simulink model "sampleModel281"  (R2021b)
settings: Solver=VariableStepAuto  StartTime=0.0  StopTime=10.0  RelTol=1e-3
undefined symbols (not defined in the file or in its folder): Newton, Raphson
libraries: simulink x13, slpidlib x3
settings Model: Creator=user  LastModifiedBy=user

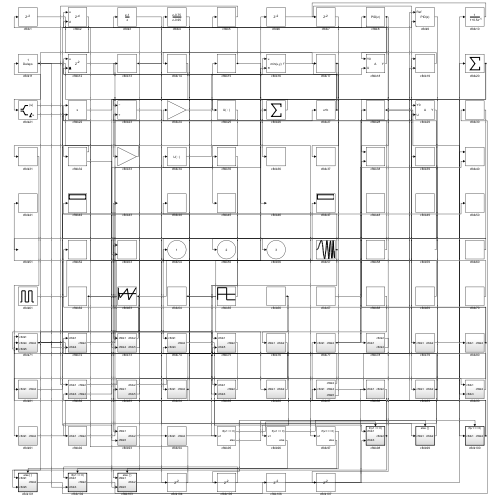
[thumbnail: Simulink's stored preview of the top-level diagram]
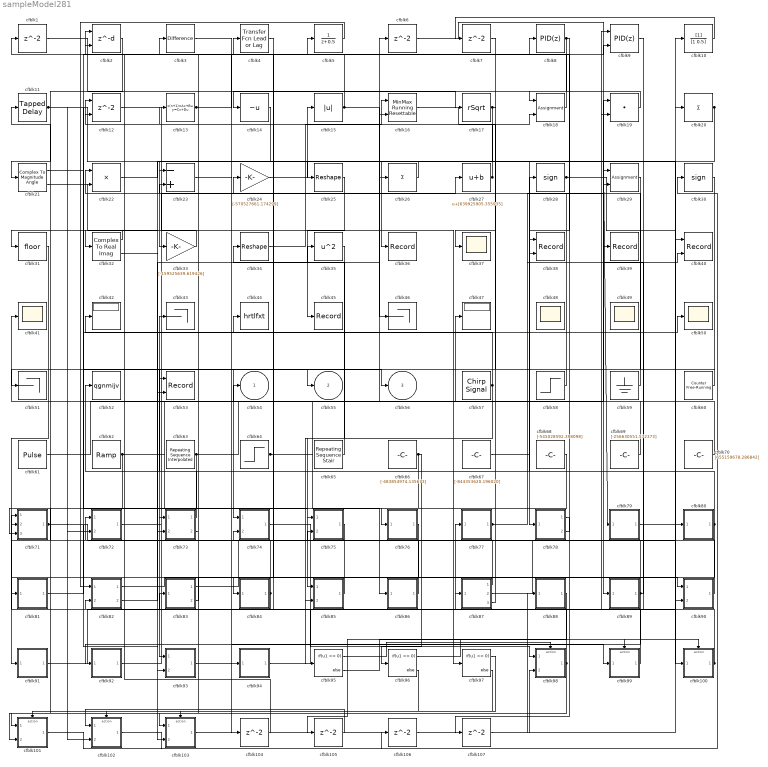
== system sampleModel281 ==
  cfblk{1,6..7,104..107} (7 alike) : Delay  SampleTime=1
  cfblk10 : DiscreteFilter  SampleTime=1
  cfblk100 : Subsystem  TreatAsAtomicUnit=on
  cfblk101 : Subsystem  TreatAsAtomicUnit=on
  cfblk102 : Subsystem  TreatAsAtomicUnit=on
  cfblk103 : Subsystem  TreatAsAtomicUnit=on
  cfblk11 : simulink/Discrete/Tapped Delay  vinit=0.0  samptime=-1  NumDelays=1  DelayOrder=Oldest  includeCurrent=off
  cfblk12 : Delay  ShowEnablePort=on  SampleTime=1
      settings: InputPortMap=u0,e6
  cfblk13 : DiscreteStateSpace
  cfblk14 : UnaryMinus
  cfblk15 : Abs
  cfblk16 : simulink/Math Operations/MinMax Running Resettable  Function=min  vinit=0.0
  cfblk17 : Sqrt  Operator=rSqrt  AlgorithmType=Newton-Raphson  SaturateOnIntegerOverflow=on
  cfblk18 : Assignment  DiagnosticForDimensions=Warning  IndexOptions=Index vector (dialog)  Indices=1  OutputSizes=1
  cfblk19 : DotProduct  InputSameDT=on  OutDataTypeStr=Inherit: Inherit via internal rule
  cfblk2 : Delay  DelayLengthSource=Input port  SampleTime=1
      settings: InputPortMap=u0,p1
  cfblk20 : Sum  Inputs=+
  cfblk21 : ComplexToMagnitudeAngle
  cfblk22 : Product  Inputs=**
  cfblk23 : Sum  Inputs=-+
  cfblk24 : Gain  Gain=[-570527661.174299]
  cfblk25 : Reshape
  cfblk26 : Sum  Inputs=+
  cfblk27 : Bias  Bias=[639925905.355935]
  cfblk28 : Signum
  cfblk29 : Assignment  DiagnosticForDimensions=Warning  IndexOptions=Index vector (dialog)  Indices=1  OutputSizes=1
  cfblk3 : simulink/Discrete/Difference  ICPrevInput=0.0  OutMin=[]  OutMax=[]  OutDataTypeStr=Inherit: Inherit via back propagation  OutDataType=fixdt(1, 16)  OutScaling=2^-10  DoSatur=off
  cfblk30 : Signum
  cfblk31 : Rounding
  cfblk32 : ComplexToRealImag
  cfblk33 : Gain  Gain=[-159525639.619426]
  cfblk34 : Reshape
  cfblk35 : Math  Operator=square  SaturateOnIntegerOverflow=on
  cfblk36 : Record  FileSettingsInternal="{\"entries\":[{\"content\":{\"excelSettings\":{\"content\":{},\"type\":\"Streamout.ExcelSettings\"}},\"type\":\"Streamout.FileSettingStorage\",\"uuid\":\"c781cdf7-8340-408b-8422-f8d69e560093\"}],\"packageUris\":[\"http://schema.mathworks.com/mf0/streamout_blocks/R2020a\"],\"version\":\"1.0\"}"  SignalsInternal="{\"entries\":[{\"content\":{\"signals\":[{\"content\":{\"blockPath\":[\"sampleModel281/cfblk36\"],\"channel\":[],\"dimensions\":[1],\"domain\":\"sampleModel281/cfblk36\",\"lineColor\":\"#139fff\",\"plots\":[1],\"port\":1,\"sid\":[\"\"],\"signalID\":11991,\"signalName\":\"cfblk17\"},\"type\":\"RecordBlkView.Signal\",\"uuid\":\"6f29a3cb-49ad-40a3-998c-ead64aca4211\"}]},\"type\":\"RecordBlkView.InputSignals\",\"uuid\":\"da20b184-1727-445b-b2e6-5f57a6227382\"}],\"packageUris\":[\"http://schema.mathworks.com/mf0/streamout_blocks/R2020a\"],\"version\":\"1.0\"}"  VisualizationBindings="{\"sparklinesplugin\":{\"info\":[{\"bindingParametersList\":[],\"subplotID\":1}]}}"
  cfblk{37,41,48..50} (5 alike) : Scope
      cfblk48 settings: Floating=on
      cfblk49 settings: Floating=on
  cfblk38 : Record  FileSettingsInternal="{\"entries\":[{\"content\":{\"excelSettings\":{\"content\":{},\"type\":\"Streamout.ExcelSettings\"}},\"type\":\"Streamout.FileSettingStorage\",\"uuid\":\"4188593c-7763-4c79-a663-ea53f92952dd\"}],\"packageUris\":[\"http://schema.mathworks.com/mf0/streamout_blocks/R2020a\"],\"version\":\"1.0\"}"  Layout=[1 1]  SignalsInternal="{\"entries\":[{\"content\":{\"signals\":[{\"content\":{\"blockPath\":[\"sampleModel281/cfblk38\"],\"channel\":[],\"dimensions\":[1],\"domain\":\"sampleModel281/cfblk38\",\"lineColor\":\"#a2142f\",\"plots\":[1],\"port\":1,\"sid\":[\"\"],\"signalID\":11963,\"signalName\":\"cfblk8\"},\"type\":\"RecordBlkView.Signal\",\"uuid\":\"ce15c6e9-b25a-4a9d-a87d-16814ede9b87\"},{\"content\":{\"blockPath\":[\"sampleModel281/cfblk38\"],\"channel\":[],\"dimensions\":[1],\"domain\":\"sampleModel281/cfblk38\",\"lineColor\":\"#139fff\",\"plots\":[1],\"port\":2,\"sid\":[\"\"],\"signalID\":11967,\"signalName\":\"cfblk80\"},\"type\":\"RecordBlkView.Signal\",\"uuid\":\"4c2adb0f-b2cf-481c-9f3f-668d91455d88\"}]},\"type\":\"RecordBlkView.InputSignals\",\"uuid\":\"ebf02ba3-550e-4026-a02e-bf4ccdc05b99\"}],\"packageUris\":[\"http://schema.mathworks.com/mf0/streamout_blocks/R2020a\"],\"version\":\"1.0\"}"  VisualizationBindings="{\"xyplotplugin\":{\"info\":[{\"series\":[{\"bindingParametersList\":[{\"parameter\":\"X-Axis\",\"signalID\":11963,\"signalName\":\"cfblk8\"},{\"parameter\":\"Y-Axis\",\"signalID\":11967,\"signalName\":\"cfblk80\"}],\"seriesID\":6983}],\"subplotID\":1}]}}"  CompatibilityTag=XY
  cfblk39 : Record  FileSettingsInternal="{\"entries\":[{\"content\":{\"excelSettings\":{\"content\":{},\"type\":\"Streamout.ExcelSettings\"}},\"type\":\"Streamout.FileSettingStorage\",\"uuid\":\"219db649-d65c-4cc3-812d-aced4d92e676\"}],\"packageUris\":[\"http://schema.mathworks.com/mf0/streamout_blocks/R2020a\"],\"version\":\"1.0\"}"  SignalsInternal="{\"entries\":[{\"content\":{\"signals\":[{\"content\":{\"blockPath\":[\"sampleModel281/cfblk39\"],\"channel\":[],\"dimensions\":[1],\"domain\":\"sampleModel281/cfblk39\",\"lineColor\":\"#edb120\",\"plots\":[1],\"port\":1,\"sid\":[\"\"],\"signalID\":11971,\"signalName\":\"cfblk89\"},\"type\":\"RecordBlkView.Signal\",\"uuid\":\"55bd96a2-e860-4ecd-af7d-bb83553d0170\"}]},\"type\":\"RecordBlkView.InputSignals\",\"uuid\":\"8836e843-c683-4200-9918-d583b1163d7b\"}],\"packageUris\":[\"http://schema.mathworks.com/mf0/streamout_blocks/R2020a\"],\"version\":\"1.0\"}"  VisualizationBindings="{\"sparklinesplugin\":{\"info\":[{\"bindingParametersList\":[],\"subplotID\":1}]}}"
  cfblk4 : simulink/Discrete/Transfer Fcn Lead or Lag  PoleZ=0.95  ZeroZ=0.75  ICPrevOutput=0.0  ICPrevInput=0.0  DoSatur=off
      settings: SourceProductBaseCode=SL
  cfblk40 : Record  FileSettingsInternal="{\"entries\":[{\"content\":{\"excelSettings\":{\"content\":{},\"type\":\"Streamout.ExcelSettings\"}},\"type\":\"Streamout.FileSettingStorage\",\"uuid\":\"7e2a92c3-6fd6-43f3-bb8d-8e942b6776ba\"}],\"packageUris\":[\"http://schema.mathworks.com/mf0/streamout_blocks/R2020a\"],\"version\":\"1.0\"}"  Layout=[1 1]  SignalsInternal="{\"entries\":[{\"content\":{\"signals\":[{\"content\":{\"blockPath\":[\"sampleModel281/cfblk40\"],\"channel\":[],\"dimensions\":[1],\"domain\":\"sampleModel281/cfblk40\",\"lineColor\":\"#a2142f\",\"plots\":[1],\"port\":1,\"sid\":[\"\"],\"signalID\":11975,\"signalName\":\"cfblk91\"},\"type\":\"RecordBlkView.Signal\",\"uuid\":\"8dd85c33-c0e1-47fe-82f9-e8373d55203a\"},{\"content\":{\"blockPath\":[\"sampleModel281/cfblk40\"],\"channel\":[],\"dimensions\":[1],\"domain\":\"sampleModel281/cfblk40\",\"lineColor\":\"#139fff\",\"plots\":[1],\"port\":2,\"sid\":[\"\"],\"signalID\":11979,\"signalName\":\"cfblk77\"},\"type\":\"RecordBlkView.Signal\",\"uuid\":\"2f79c080-1485-4a3a-9cf0-de9ca85e6d7b\"}]},\"type\":\"RecordBlkView.InputSignals\",\"uuid\":\"15f4dd09-4716-4c1b-9d4f-630d21f687a7\"}],\"packageUris\":[\"http://schema.mathworks.com/mf0/streamout_blocks/R2020a\"],\"version\":\"1.0\"}"  VisualizationBindings="{\"xyplotplugin\":{\"info\":[{\"series\":[{\"bindingParametersList\":[{\"parameter\":\"X-Axis\",\"signalID\":11975,\"signalName\":\"cfblk91\"},{\"parameter\":\"Y-Axis\",\"signalID\":11979,\"signalName\":\"cfblk77\"}],\"seriesID\":59243}],\"subplotID\":1}]}}"  CompatibilityTag=XY
  cfblk42 : Display
  cfblk43 : Terminator
  cfblk44 : ToWorkspace  VariableName=hrtlfxt  SaveFormat=Timeseries  SampleTime=-1
  cfblk45 : Record  FileSettingsInternal="{\"entries\":[{\"content\":{\"excelSettings\":{\"content\":{},\"type\":\"Streamout.ExcelSettings\"}},\"type\":\"Streamout.FileSettingStorage\",\"uuid\":\"80b63704-7d10-486e-b387-18bfb6728c18\"}],\"packageUris\":[\"http://schema.mathworks.com/mf0/streamout_blocks/R2020a\"],\"version\":\"1.0\"}"  SignalsInternal="{\"entries\":[{\"content\":{\"signals\":[{\"content\":{\"blockPath\":[\"sampleModel281/cfblk45\"],\"channel\":[],\"dimensions\":[1],\"domain\":\"sampleModel281/cfblk45\",\"lineColor\":\"#ff6929\",\"plots\":[1],\"port\":1,\"sid\":[\"\"],\"signalID\":11995,\"signalName\":\"cfblk25\"},\"type\":\"RecordBlkView.Signal\",\"uuid\":\"f8ece178-e086-4969-b784-ed276f630d12\"}]},\"type\":\"RecordBlkView.InputSignals\",\"uuid\":\"7be7d227-b162-4c4c-ad33-f79b945d64e0\"}],\"packageUris\":[\"http://schema.mathworks.com/mf0/streamout_blocks/R2020a\"],\"version\":\"1.0\"}"  VisualizationBindings="{\"sparklinesplugin\":{\"info\":[{\"bindingParametersList\":[],\"subplotID\":1}]}}"
  cfblk46 : Terminator
  cfblk47 : Display
  cfblk5 : DiscreteTransferFcn  SampleTime=1
  cfblk51 : Terminator
  cfblk52 : ToWorkspace  VariableName=qgnmijv  SaveFormat=Timeseries  SampleTime=-1
  cfblk53 : Record  FileSettingsInternal="{\"entries\":[{\"content\":{\"excelSettings\":{\"content\":{},\"type\":\"Streamout.ExcelSettings\"}},\"type\":\"Streamout.FileSettingStorage\",\"uuid\":\"979e6c69-9637-4301-9808-cdf47ec4f26d\"}],\"packageUris\":[\"http://schema.mathworks.com/mf0/streamout_blocks/R2020a\"],\"version\":\"1.0\"}"  Layout=[1 1]  SignalsInternal="{\"entries\":[{\"content\":{\"signals\":[{\"content\":{\"blockPath\":[\"sampleModel281/cfblk53\"],\"channel\":[],\"dimensions\":[1],\"domain\":\"sampleModel281/cfblk53\",\"lineColor\":\"#a2142f\",\"plots\":[1],\"port\":1,\"sid\":[\"\"],\"signalID\":11983,\"signalName\":\"cfblk86\"},\"type\":\"RecordBlkView.Signal\",\"uuid\":\"a6416475-d9fb-464a-9363-37660f0059bb\"},{\"content\":{\"blockPath\":[\"sampleModel281/cfblk53\"],\"channel\":[],\"dimensions\":[1],\"domain\":\"sampleModel281/cfblk53\",\"lineColor\":\"#139fff\",\"plots\":[1],\"port\":2,\"sid\":[\"\"],\"signalID\":11987,\"signalName\":\"cfblk21:2\"},\"type\":\"RecordBlkView.Signal\",\"uuid\":\"573ba67e-6b02-4113-b266-649fc294594e\"}]},\"type\":\"RecordBlkView.InputSignals\",\"uuid\":\"a6bf4982-741b-4a82-8cf7-86aa072de18b\"}],\"packageUris\":[\"http://schema.mathworks.com/mf0/streamout_blocks/R2020a\"],\"version\":\"1.0\"}"  VisualizationBindings="{\"xyplotplugin\":{\"info\":[{\"series\":[{\"bindingParametersList\":[{\"parameter\":\"X-Axis\",\"signalID\":11983,\"signalName\":\"cfblk86\"},{\"parameter\":\"Y-Axis\",\"signalID\":11987,\"signalName\":\"cfblk21:2\"}],\"seriesID\":45068}],\"subplotID\":1}]}}"  CompatibilityTag=XY
  cfblk57 : simulink/Sources/Chirp Signal  f1=[-334643469.224714]  T=[-94135203.309986]  f2=[152847106.360706]
  cfblk58 : Step  Time=[42.000000]  Before=[-159427746.311310]  After=[840646586.279118]  SampleTime=0
  cfblk59 : Ground
  cfblk60 : simulink/Sources/Counter Free-Running  NumBits=[16.000000]  tsamp=-1
  cfblk61 : DiscretePulseGenerator  PulseType=Time based  Amplitude=[-599555559.374941]  Period=[82024512.109082]  PulseWidth=5  PhaseDelay=[9.000000]
  cfblk62 : simulink/Sources/Ramp  slope=[-4599.343733]  start=[27.677113]  InitialOutput=[-405546.025741]
  cfblk63 : simulink/Sources/Repeating Sequence Interpolated  OutValues=[236426282.621736, -510010552.768380, 614187584.766331, -765152925.585290, 735747006.586161]  TimeValues=[0 0.1 0.5 0.6 1].'  LookUpMeth=Use Input Below  tsamp=0.01  OutMin=[]  OutMax=[]  OutDataTypeStr=double  OutputDataTypeScalingMode=double  OutDataType=fixdt(0,8)  OutScaling=2^-10
  cfblk64 : Step  Time=[34.000000]  Before=[-566169938.934532]  After=[306635443.375634]  SampleTime=0
  cfblk65 : simulink/Sources/Repeating Sequence Stair  OutValues=[982481802.198341, -856880890.360256]  tsamp=-1  OutMin=[]  OutMax=[]  OutDataTypeStr=double  OutputDataTypeScalingMode=double  OutDataType=fixdt(0,8)  ConRadixGroup=Best Precision: Vector-wise  OutScaling=2^-12
  cfblk66 : Constant  Value=[-483854974.135673]  SampleTime=1
  cfblk67 : Constant  Value=[-844353620.196020]  SampleTime=1
  cfblk68 : Constant  Value=[-545028592.398098]  SampleTime=1
  cfblk69 : Constant  Value=[-256630551.572373]  SampleTime=1
  cfblk70 : Constant  Value=[655159678.286842]  SampleTime=1
  cfblk71 : Subsystem
  cfblk72 : Subsystem
  cfblk73 : Subsystem
  cfblk74 : Subsystem
  cfblk75 : Subsystem
  cfblk76 : Subsystem
  cfblk77 : Subsystem
  cfblk78 : Subsystem
  cfblk79 : Subsystem
  cfblk8 : slpidlib/PID Controller  Controller=PID  Form=Parallel  TimeDomain=Discrete-time  UseExternalTs=off  SampleTime=1  IntegratorMethod=Forward Euler  FilterMethod=Forward Euler  ControllerParametersSource=internal  P=1  I=1  D=0  UseFilter=on  N=100  TunerSelectOption=Transfer Function Based (PID Tuner App)  InitialConditionSource=internal  InitialConditionForIntegrator=0  InitialConditionForFilter=0  DifferentiatorICPrevScaledInput=0  ExternalReset=none  TrackingMode=off  Kt=1  LimitOutput=off  SatLimitsSource=internal  UpperSaturationLimit=inf  LowerSaturationLimit=-inf  LinearizeAsGain=off  AntiWindupMode=none  Kb=1  POutMin=[]  POutMax=[]  IOutMin=[]  IOutMax=[]  DOutMin=[]  DOutMax=[]  NOutMin=[]  NOutMax=[]  SumOutMin=[]  SumOutMax=[]  SaturationOutMin=[]  SaturationOutMax=[]  PParamMin=[]  PParamMax=[]  IParamMin=[]  IParamMax=[]  DParamMin=[]  DParamMax=[]  NParamMin=[]  NParamMax=[]  KbParamMin=[]  KbParamMax=[]  KtParamMin=[]  KtParamMax=[]  KbOutMin=[]  KbOutMax=[]  KtOutMin=[]  KtOutMax=[]  IntegratorOutMin=[]  IntegratorOutMax=[]  FilterOutMin=[]  FilterOutMax=[]  SumI1OutMin=[]  SumI1OutMax=[]  SumI2OutMin=[]  SumI2OutMax=[]  SumI3OutMin=[]  SumI3OutMax=[]  SumI4OutMin=[]  SumI4OutMax=[]  SumDOutMin=[]  SumDOutMax=[]  DifferentiatorOutMin=[]  DifferentiatorOutMax=[]  FilterDiffOutCoefMin=[]  FilterDiffOutCoefMax=[]  ReciprocalOutMin=[]  ReciprocalOutMax=[]  SumDenOutMin=[]  SumDenOutMax=[]  SumNumOutMin=[]  SumNumOutMax=[]  DivideOutMin=[]  DivideOutMax=[]  UdiffTsProdOutMin=[]  UdiffTsProdOutMax=[]  NTsProdOutMin=[]  NTsProdOutMax=[]  UintegralTsProdOutMin=[]  UintegralTsProdOutMax=[]  UngainTsProdOutMin=[]  UngainTsProdOutMax=[]  IntegratorContinuousStateAttributes=''  IntegratorStateMustResolveToSignalObject=off  IntegratorRTWStateStorageClass=Auto  FilterContinuousStateAttributes=''  FilterStateMustResolveToSignalObject=off  FilterRTWStateStorageClass=Auto  ParallelPVariant=InternalParameters  IdealPVariant=Disabled  IVariant=InternalParameters  DVariant=InternalParameters  IntegratorVariant=Discrete  SatVariant=Disabled  AWVariant=Passthrough  PCopyVariant=Disabled  TRVariant=Disabled  FdbkBlocksVariant=Forward  IdealPFdbkVariant=Disabled  SatFdbkVariant=Disabled  DerivativeFilterVariant=ForwardEulerFilter  NVariant=InternalParameters  NCopyVariant=Disabled  FilterICVariant=InternalICsFilter  IntegratorICVariant=InternalICs  ExternalResetVariant=Disabled  TRSumVariant=Passthrough  SumFdbkVariant=Disabled  SumVariant=Sum_PID  TsampFilterVariant=InternalTs  TsampNgainVariant=Passthrough  TsampIntegralVariant=Passthrough  ExternalSaturationOutDataTypeStr=Inherit: Same as second input
  cfblk80 : Subsystem
  cfblk81 : Subsystem
  cfblk82 : Subsystem
  cfblk83 : Subsystem
  cfblk84 : Subsystem
  cfblk85 : Subsystem
  cfblk86 : Subsystem
  cfblk87 : Subsystem
  cfblk88 : Subsystem
  cfblk89 : Subsystem
  cfblk9 : slpidlib/PID Controller (2DOF)  Controller=PID  Form=Parallel  TimeDomain=Discrete-time  UseExternalTs=off  SampleTime=1  IntegratorMethod=Forward Euler  FilterMethod=Forward Euler  ControllerParametersSource=internal  P=1  I=1  D=0  UseFilter=on  N=100  b=1  c=1  TunerSelectOption=Transfer Function Based (PID Tuner App)  InitialConditionSource=internal  InitialConditionForIntegrator=0  InitialConditionForFilter=0  DifferentiatorICPrevScaledInput=0  ExternalReset=none  TrackingMode=off  Kt=1  LimitOutput=off  SatLimitsSource=internal  UpperSaturationLimit=inf  LowerSaturationLimit=-inf  LinearizeAsGain=off  AntiWindupMode=none  Kb=1  POutMin=[]  POutMax=[]  IOutMin=[]  IOutMax=[]  DOutMin=[]  DOutMax=[]  NOutMin=[]  NOutMax=[]  bOutMin=[]  bOutMax=[]  cOutMin=[]  cOutMax=[]  SumOutMin=[]  SumOutMax=[]  SaturationOutMin=[]  SaturationOutMax=[]  PParamMin=[]  PParamMax=[]  IParamMin=[]  IParamMax=[]  DParamMin=[]  DParamMax=[]  NParamMin=[]  NParamMax=[]  bParamMin=[]  bParamMax=[]  cParamMin=[]  cParamMax=[]  KbParamMin=[]  KbParamMax=[]  KtParamMin=[]  KtParamMax=[]  KbOutMin=[]  KbOutMax=[]  KtOutMin=[]  KtOutMax=[]  IntegratorOutMin=[]  IntegratorOutMax=[]  FilterOutMin=[]  FilterOutMax=[]  SumI1OutMin=[]  SumI1OutMax=[]  SumI2OutMin=[]  SumI2OutMax=[]  SumI3OutMin=[]  SumI3OutMax=[]  SumI4OutMin=[]  SumI4OutMax=[]  SumDOutMin=[]  SumDOutMax=[]  Sum1OutMin=[]  Sum1OutMax=[]  Sum2OutMin=[]  Sum2OutMax=[]  Sum3OutMin=[]  Sum3OutMax=[]  DifferentiatorOutMin=[]  DifferentiatorOutMax=[]  FilterDiffOutCoefMin=[]  FilterDiffOutCoefMax=[]  ReciprocalOutMin=[]  ReciprocalOutMax=[]  SumDenOutMin=[]  SumDenOutMax=[]  SumNumOutMin=[]  SumNumOutMax=[]  DivideOutMin=[]  DivideOutMax=[]  UdiffTsProdOutMin=[]  UdiffTsProdOutMax=[]  NTsProdOutMin=[]  NTsProdOutMax=[]  UintegralTsProdOutMin=[]  UintegralTsProdOutMax=[]  UngainTsProdOutMin=[]  UngainTsProdOutMax=[]  IntegratorContinuousStateAttributes=''  IntegratorStateMustResolveToSignalObject=off  IntegratorRTWStateStorageClass=Auto  FilterContinuousStateAttributes=''  FilterStateMustResolveToSignalObject=off  FilterRTWStateStorageClass=Auto  ParallelPVariant=InternalParameters  IdealPVariant=Disabled  IVariant=InternalParameters  DVariant=InternalParameters  bVariant=InternalParameters  cVariant=InternalParameters  IntegratorVariant=Discrete  SatVariant=Disabled  AWVariant=Passthrough  PCopyVariant=Disabled  TRVariant=Disabled  FdbkBlocksVariant=Forward  IdealPFdbkVariant=Disabled  SatFdbkVariant=Disabled  DerivativeFilterVariant=ForwardEulerFilter  NVariant=InternalParameters  NCopyVariant=Disabled  FilterICVariant=InternalICsFilter  IntegratorICVariant=InternalICs  ExternalResetVariant=Disabled  TRSumVariant=Passthrough  SumFdbkVariant=Disabled  SumVariant=Sum_PID  TsampFilterVariant=InternalTs  TsampNgainVariant=Passthrough  TsampIntegralVariant=Passthrough  ExternalSaturationOutDataTypeStr=Inherit: Same as second input
      settings: SourceProductBaseCode=SL
  cfblk90 : Subsystem
  cfblk91 : Subsystem
  cfblk92 : Subsystem
  cfblk93 : Subsystem
  cfblk94 : Subsystem
  cfblk95 : If  IfExpression=u1 >= 0  SampleTime=1
  cfblk96 : If  IfExpression=u1 >= 0  SampleTime=1
  cfblk97 : If  IfExpression=u1 >= 0  SampleTime=1
  cfblk98 : Subsystem  TreatAsAtomicUnit=on
  cfblk99 : Subsystem  TreatAsAtomicUnit=on
  cfblk54 : Outport
  cfblk55 : Outport  Port=2
  cfblk56 : Outport  Port=3
  wires:
  cfblk92/1(cfblk2) -> cfblk27/1
  cfblk7/1 -> cfblk55/1
  cfblk17/1 -> cfblk36/1, cfblk37/1
  cfblk14/1 -> cfblk33/1
  cfblk58/1 -> cfblk24/1
  cfblk57/1 -> cfblk42/1, cfblk85/2(cfblk3)
  cfblk6/1 -> cfblk89/1(cfblk1)
  cfblk72/1(cfblk2) -> cfblk26/1
  cfblk65/1 -> cfblk4/1
  cfblk76/1(cfblk2) -> cfblk103/1(cfblk1)
  cfblk9/1 -> cfblk77/1(cfblk1)
  cfblk4/1 -> cfblk84/1(cfblk1)
  cfblk31/1 -> cfblk91/1(cfblk1)
  cfblk25/1 -> cfblk45/1
  cfblk19/1 -> cfblk18/1
  cfblk29/1 -> cfblk74/1(cfblk1)
  cfblk33/1 -> cfblk32/1
  cfblk100/1(cfblk2) -> cfblk54/1, cfblk71/2(cfblk4)
  cfblk28/1 -> cfblk79/1(cfblk1), cfblk90/2(cfblk3)
  cfblk5/1 -> cfblk82/1(cfblk1)
  cfblk70/1 -> cfblk41/1
  cfblk66/1 -> cfblk76/1(cfblk1), cfblk96/1
  cfblk20/1 -> cfblk78/1(cfblk1), cfblk103/2(cfblk5)
  cfblk60/1 -> cfblk51/1
  cfblk16/1 -> cfblk18/2
  cfblk75/1(cfblk2) -> cfblk74/2(cfblk3)
  cfblk8/1 -> cfblk14/1, cfblk38/1
  cfblk102/1(cfblk2) -> cfblk30/1
  cfblk12/1 -> cfblk97/1
  cfblk74/1(cfblk2) -> cfblk98/1(cfblk1)
  cfblk30/1 -> cfblk93/1(cfblk1)
  cfblk98/1(cfblk2) -> cfblk87/1(cfblk1), cfblk101/2(cfblk5)
  cfblk87/1(cfblk2) -> cfblk44/1
  cfblk68/1 -> cfblk73/1(cfblk1)
  cfblk26/1 -> cfblk23/1
  cfblk35/1 -> cfblk85/1(cfblk1)
  cfblk61/1 -> cfblk19/1
  cfblk90/1(cfblk2) -> cfblk11/1
  cfblk15/1 -> cfblk46/1, cfblk1/1
  cfblk1/1 -> cfblk17/1
  cfblk82/1(cfblk2) -> cfblk90/1(cfblk1)
  cfblk80/1(cfblk2) -> cfblk52/1, cfblk38/2, cfblk81/1(cfblk1)
  cfblk69/1 -> cfblk22/1
  cfblk73/1(cfblk2) -> cfblk43/1
  cfblk84/1(cfblk2) -> cfblk13/1, cfblk82/2(cfblk3)
  cfblk86/1(cfblk2) -> cfblk53/1
  cfblk11/1 -> cfblk100/1(cfblk1), cfblk72/2(cfblk4), cfblk56/1
  cfblk87/2(cfblk4) -> cfblk10/1
  cfblk73/2(cfblk5) -> cfblk23/2
  cfblk2/1 -> cfblk21/1
  cfblk23/1 -> cfblk94/1(cfblk1)
  cfblk89/1(cfblk2) -> cfblk39/1, cfblk34/1, cfblk92/1(cfblk1)
  cfblk18/1 -> cfblk2/1
  cfblk10/1 -> cfblk7/1
  cfblk64/1 -> cfblk86/1(cfblk1), cfblk47/1
  cfblk24/1 -> cfblk15/1
  cfblk79/1(cfblk2) -> cfblk80/1(cfblk1)
  cfblk99/1(cfblk2) -> cfblk83/1(cfblk1)
  cfblk83/1(cfblk2) -> cfblk9/1
  cfblk94/1(cfblk2) -> cfblk19/2
  cfblk21/1 -> cfblk75/1(cfblk1)
  cfblk3/1 -> cfblk99/1(cfblk1)
  cfblk82/2(cfblk4) -> cfblk35/1
  cfblk34/1 -> cfblk16/1
  cfblk71/1(cfblk2) -> cfblk75/2(cfblk5), cfblk93/2(cfblk5), cfblk102/2(cfblk3), cfblk50/1
  cfblk85/1(cfblk2) -> cfblk71/1(cfblk1)
  cfblk103/1(cfblk2) -> cfblk88/1(cfblk1)
  cfblk62/1 -> cfblk95/1, cfblk16/2, cfblk101/1(cfblk1)
  cfblk22/1 -> cfblk25/1
  cfblk81/1(cfblk2) -> cfblk8/1
  cfblk83/2(cfblk5) -> cfblk72/1(cfblk1)
  cfblk21/2 -> cfblk53/2
  cfblk63/1 -> cfblk6/1, cfblk71/3(cfblk5)
  cfblk91/1(cfblk2) -> cfblk40/1
  cfblk13/1 -> cfblk9/2, cfblk29/1
  cfblk87/3(cfblk5) -> cfblk12/1
  cfblk78/2(cfblk4) -> cfblk5/1
  cfblk67/1 -> cfblk28/1
  cfblk27/1 -> cfblk12/2, cfblk3/1
  cfblk77/1(cfblk2) -> cfblk40/2, cfblk29/2
  cfblk32/1 -> cfblk31/1
  cfblk59/1 -> cfblk22/2
  cfblk32/2 -> cfblk73/2(cfblk4)
  cfblk95/1 -> cfblk98/Action
  cfblk95/2 -> cfblk99/Action
  cfblk96/1 -> cfblk100/Action
  cfblk96/2 -> cfblk101/Action
  cfblk97/1 -> cfblk102/Action
  cfblk97/2 -> cfblk103/Action
  cfblk93/1(cfblk2) -> cfblk104/1
  cfblk104/1 -> cfblk2/2
  cfblk88/1(cfblk2) -> cfblk105/1
  cfblk105/1 -> cfblk102/1(cfblk1)
  cfblk101/1(cfblk2) -> cfblk106/1
  cfblk106/1 -> cfblk98/2(cfblk3)
  cfblk78/1(cfblk2) -> cfblk107/1
  cfblk107/1 -> cfblk20/1

== system sampleModel281/cfblk100 ==
  cfblk1 : Inport
  Action Port : ActionPort  ActionPortLabel=if(u1 >= 0)
  cfblk3 : DiscreteStateSpace  SampleTime=-1
  cfblk2 : Outport
  wires:
  cfblk3/1 -> cfblk2/1
  cfblk1/1 -> cfblk3/1

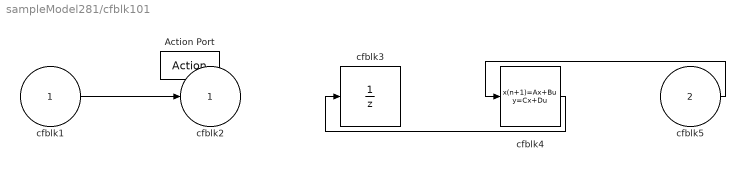
== system sampleModel281/cfblk101 ==
  cfblk1 : Inport
  cfblk5 : Inport  Port=2
  Action Port : ActionPort  ActionPortLabel=else
  cfblk3 : UnitDelay  SampleTime=-1  HasFrameUpgradeWarning=on
  cfblk4 : DiscreteStateSpace  SampleTime=-1
  cfblk2 : Outport
  wires:
  cfblk5/1 -> cfblk4/1
  cfblk4/1 -> cfblk3/1
  cfblk1/1 -> cfblk2/1

== system sampleModel281/cfblk102 ==
  cfblk1 : Inport
  cfblk3 : Inport  Port=2
  Action Port : ActionPort  ActionPortLabel=if(u1 >= 0)
  cfblk2 : Outport
  wires:
  cfblk1/1 -> cfblk2/1

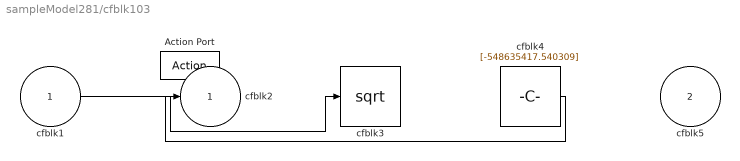
== system sampleModel281/cfblk103 ==
  cfblk1 : Inport
  cfblk5 : Inport  Port=2
  Action Port : ActionPort  ActionPortLabel=else
  cfblk3 : Sqrt  SaturateOnIntegerOverflow=on
  cfblk4 : Constant  Value=[-548635417.540309]  SampleTime=1
  cfblk2 : Outport
  wires:
  cfblk1/1 -> cfblk3/1
  cfblk4/1 -> cfblk2/1

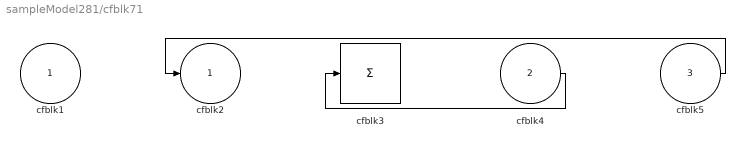
== system sampleModel281/cfblk71 ==
  cfblk1 : Inport
  cfblk4 : Inport  Port=2
  cfblk5 : Inport  Port=3
  cfblk3 : Sum  Inputs=+
  cfblk2 : Outport
  wires:
  cfblk5/1 -> cfblk2/1
  cfblk4/1 -> cfblk3/1

== system sampleModel281/cfblk72 ==
  cfblk1 : Inport
  cfblk4 : Inport  Port=2
  cfblk3 : Assignment  DiagnosticForDimensions=Warning  IndexOptions=Index vector (dialog)  Indices=1  OutputSizes=1
  cfblk2 : Outport
  wires:
  cfblk3/1 -> cfblk2/1
  cfblk1/1 -> cfblk3/1
  cfblk4/1 -> cfblk3/2

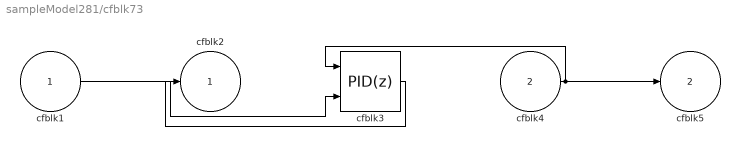
== system sampleModel281/cfblk73 ==
  cfblk1 : Inport
  cfblk4 : Inport  Port=2
  cfblk3 : slpidlib/PID Controller (2DOF)  Controller=PID  Form=Parallel  TimeDomain=Discrete-time  UseExternalTs=off  SampleTime=1  IntegratorMethod=Forward Euler  FilterMethod=Forward Euler  ControllerParametersSource=internal  P=1  I=1  D=0  UseFilter=on  N=100  b=1  c=1  TunerSelectOption=Transfer Function Based (PID Tuner App)  InitialConditionSource=internal  InitialConditionForIntegrator=0  InitialConditionForFilter=0  DifferentiatorICPrevScaledInput=0  ExternalReset=none  TrackingMode=off  Kt=1  LimitOutput=off  SatLimitsSource=internal  UpperSaturationLimit=inf  LowerSaturationLimit=-inf  LinearizeAsGain=off  AntiWindupMode=none  Kb=1  POutMin=[]  POutMax=[]  IOutMin=[]  IOutMax=[]  DOutMin=[]  DOutMax=[]  NOutMin=[]  NOutMax=[]  bOutMin=[]  bOutMax=[]  cOutMin=[]  cOutMax=[]  SumOutMin=[]  SumOutMax=[]  SaturationOutMin=[]  SaturationOutMax=[]  PParamMin=[]  PParamMax=[]  IParamMin=[]  IParamMax=[]  DParamMin=[]  DParamMax=[]  NParamMin=[]  NParamMax=[]  bParamMin=[]  bParamMax=[]  cParamMin=[]  cParamMax=[]  KbParamMin=[]  KbParamMax=[]  KtParamMin=[]  KtParamMax=[]  KbOutMin=[]  KbOutMax=[]  KtOutMin=[]  KtOutMax=[]  IntegratorOutMin=[]  IntegratorOutMax=[]  FilterOutMin=[]  FilterOutMax=[]  SumI1OutMin=[]  SumI1OutMax=[]  SumI2OutMin=[]  SumI2OutMax=[]  SumI3OutMin=[]  SumI3OutMax=[]  SumI4OutMin=[]  SumI4OutMax=[]  SumDOutMin=[]  SumDOutMax=[]  Sum1OutMin=[]  Sum1OutMax=[]  Sum2OutMin=[]  Sum2OutMax=[]  Sum3OutMin=[]  Sum3OutMax=[]  DifferentiatorOutMin=[]  DifferentiatorOutMax=[]  FilterDiffOutCoefMin=[]  FilterDiffOutCoefMax=[]  ReciprocalOutMin=[]  ReciprocalOutMax=[]  SumDenOutMin=[]  SumDenOutMax=[]  SumNumOutMin=[]  SumNumOutMax=[]  DivideOutMin=[]  DivideOutMax=[]  UdiffTsProdOutMin=[]  UdiffTsProdOutMax=[]  NTsProdOutMin=[]  NTsProdOutMax=[]  UintegralTsProdOutMin=[]  UintegralTsProdOutMax=[]  UngainTsProdOutMin=[]  UngainTsProdOutMax=[]  IntegratorContinuousStateAttributes=''  IntegratorStateMustResolveToSignalObject=off  IntegratorRTWStateStorageClass=Auto  FilterContinuousStateAttributes=''  FilterStateMustResolveToSignalObject=off  FilterRTWStateStorageClass=Auto  ParallelPVariant=InternalParameters  IdealPVariant=Disabled  IVariant=InternalParameters  DVariant=InternalParameters  bVariant=InternalParameters  cVariant=InternalParameters  IntegratorVariant=Discrete  SatVariant=Disabled  AWVariant=Passthrough  PCopyVariant=Disabled  TRVariant=Disabled  FdbkBlocksVariant=Forward  IdealPFdbkVariant=Disabled  SatFdbkVariant=Disabled  DerivativeFilterVariant=ForwardEulerFilter  NVariant=InternalParameters  NCopyVariant=Disabled  FilterICVariant=InternalICsFilter  IntegratorICVariant=InternalICs  ExternalResetVariant=Disabled  TRSumVariant=Passthrough  SumFdbkVariant=Disabled  SumVariant=Sum_PID  TsampFilterVariant=InternalTs  TsampNgainVariant=Passthrough  TsampIntegralVariant=Passthrough  ExternalSaturationOutDataTypeStr=Inherit: Same as second input
      settings: SourceProductBaseCode=SL
  cfblk2 : Outport
  cfblk5 : Outport  Port=2
  wires:
  cfblk4/1 -> cfblk3/1, cfblk5/1
  cfblk1/1 -> cfblk3/2
  cfblk3/1 -> cfblk2/1

== system sampleModel281/cfblk74 ==
  cfblk1 : Inport
  cfblk3 : Inport  Port=2
  cfblk2 : Outport
  wires:
  cfblk3/1 -> cfblk2/1

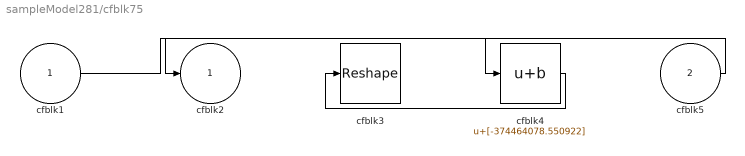
== system sampleModel281/cfblk75 ==
  cfblk1 : Inport
  cfblk5 : Inport  Port=2
  cfblk3 : Reshape
  cfblk4 : Bias  Bias=[-374464078.550922]
  cfblk2 : Outport
  wires:
  cfblk5/1 -> cfblk2/1
  cfblk4/1 -> cfblk3/1
  cfblk1/1 -> cfblk4/1

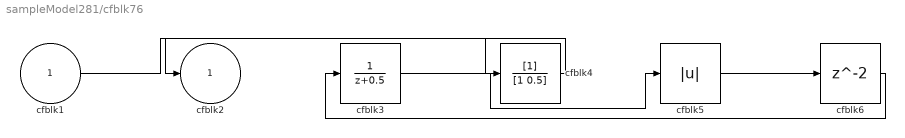
== system sampleModel281/cfblk76 ==
  cfblk1 : Inport
  cfblk3 : DiscreteTransferFcn  SampleTime=1
  cfblk4 : DiscreteFilter  SampleTime=1
  cfblk5 : Abs
  cfblk6 : Delay  SampleTime=1
  cfblk2 : Outport
  wires:
  cfblk4/1 -> cfblk2/1
  cfblk3/1 -> cfblk5/1
  cfblk1/1 -> cfblk4/1
  cfblk5/1 -> cfblk6/1
  cfblk6/1 -> cfblk3/1

== system sampleModel281/cfblk77 ==
  cfblk1 : Inport
  cfblk3 : simulink/Math Operations/MinMax Running Resettable  Function=min  vinit=0.0
  cfblk2 : Outport
  wires:
  cfblk1/1 -> cfblk3/1, cfblk3/2
  cfblk3/1 -> cfblk2/1

== system sampleModel281/cfblk78 ==
  cfblk1 : Inport
  cfblk3 : simulink/Discrete/Difference  ICPrevInput=0.0  OutMin=[]  OutMax=[]  OutDataTypeStr=Inherit: Inherit via back propagation  OutDataType=fixdt(1, 16)  OutScaling=2^-10  DoSatur=off
  cfblk2 : Outport
  cfblk4 : Outport  Port=2
  wires:
  cfblk1/1 -> cfblk4/1, cfblk3/1
  cfblk3/1 -> cfblk2/1

== system sampleModel281/cfblk79 ==
  cfblk1 : Inport
  cfblk3 : Gain  Gain=[-540929469.649708]
  cfblk4 : Constant  Value=[345199688.545486]  SampleTime=1
  cfblk2 : Outport
  wires:
  cfblk4/1 -> cfblk3/1
  cfblk1/1 -> cfblk2/1

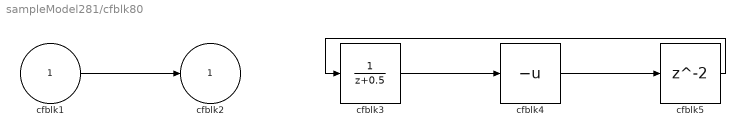
== system sampleModel281/cfblk80 ==
  cfblk1 : Inport
  cfblk3 : DiscreteTransferFcn  SampleTime=1
  cfblk4 : UnaryMinus
  cfblk5 : Delay  SampleTime=1
  cfblk2 : Outport
  wires:
  cfblk1/1 -> cfblk2/1
  cfblk3/1 -> cfblk4/1
  cfblk4/1 -> cfblk5/1
  cfblk5/1 -> cfblk3/1

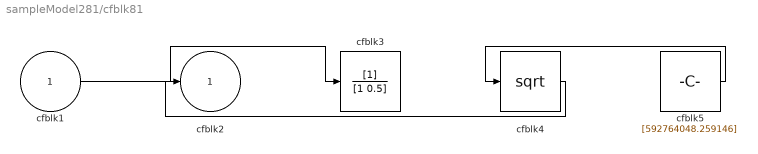
== system sampleModel281/cfblk81 ==
  cfblk1 : Inport
  cfblk3 : DiscreteFilter  SampleTime=1
  cfblk4 : Sqrt  SaturateOnIntegerOverflow=on
  cfblk5 : Constant  Value=[592764048.259146]  SampleTime=1
  cfblk2 : Outport
  wires:
  cfblk1/1 -> cfblk3/1
  cfblk4/1 -> cfblk2/1
  cfblk5/1 -> cfblk4/1

== system sampleModel281/cfblk82 ==
  cfblk1 : Inport
  cfblk3 : Inport  Port=2
  cfblk2 : Outport
  cfblk4 : Outport  Port=2
  wires:
  cfblk1/1 -> cfblk2/1
  cfblk3/1 -> cfblk4/1

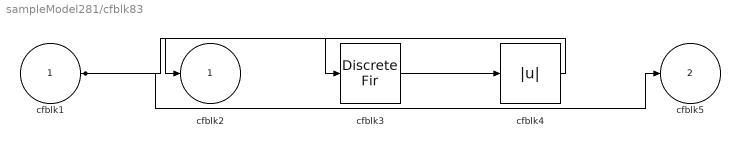
== system sampleModel281/cfblk83 ==
  cfblk1 : Inport
  cfblk3 : DiscreteFir  SampleTime=1
  cfblk4 : Abs
  cfblk2 : Outport
  cfblk5 : Outport  Port=2
  wires:
  cfblk4/1 -> cfblk2/1
  cfblk3/1 -> cfblk4/1
  cfblk1/1 -> cfblk5/1, cfblk3/1

== system sampleModel281/cfblk84 ==
  cfblk1 : Inport
  cfblk3 : UnitDelay  HasFrameUpgradeWarning=on
  cfblk2 : Outport
  wires:
  cfblk1/1 -> cfblk3/1
  cfblk3/1 -> cfblk2/1

== system sampleModel281/cfblk85 ==
  cfblk1 : Inport
  cfblk3 : Inport  Port=2
  cfblk2 : Outport
  wires:
  cfblk1/1 -> cfblk2/1

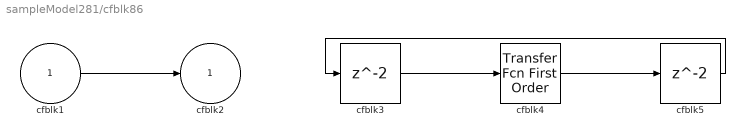
== system sampleModel281/cfblk86 ==
  cfblk1 : Inport
  cfblk3 : Delay  SampleTime=1
  cfblk4 : simulink/Discrete/Transfer Fcn First Order  PoleZ=0.95  ICPrevOutput=0.0  DoSatur=off
  cfblk5 : Delay  SampleTime=1
  cfblk2 : Outport
  wires:
  cfblk3/1 -> cfblk4/1
  cfblk1/1 -> cfblk2/1
  cfblk4/1 -> cfblk5/1
  cfblk5/1 -> cfblk3/1

== system sampleModel281/cfblk87 ==
  cfblk1 : Inport
  cfblk3 : simulink/Math Operations/MinMax Running Resettable  Function=min  vinit=0.0
  cfblk2 : Outport
  cfblk4 : Outport  Port=2
  cfblk5 : Outport  Port=3
  wires:
  cfblk3/1 -> cfblk2/1, cfblk5/1
  cfblk1/1 -> cfblk4/1, cfblk3/1, cfblk3/2

== system sampleModel281/cfblk88 ==
  cfblk1 : Inport
  cfblk3 : Delay  DelayLengthSource=Input port  SampleTime=1
      settings: InputPortMap=u0,p1
  cfblk4 : Sqrt  Operator=rSqrt  AlgorithmType=Newton-Raphson  SaturateOnIntegerOverflow=on
  cfblk5 : UnaryMinus
  cfblk2 : Outport
  wires:
  cfblk1/1 -> cfblk3/1, cfblk5/1
  cfblk5/1 -> cfblk3/2
  cfblk3/1 -> cfblk4/1
  cfblk4/1 -> cfblk2/1

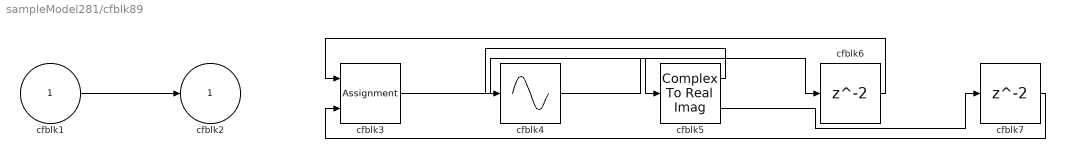
== system sampleModel281/cfblk89 ==
  cfblk1 : Inport
  cfblk3 : Assignment  DiagnosticForDimensions=Warning  IndexOptions=Index vector (dialog)  Indices=1  OutputSizes=1
  cfblk4 : Sin  TimeSource=Use external signal  SampleTime=0
  cfblk5 : ComplexToRealImag
  cfblk6 : Delay  SampleTime=1
  cfblk7 : Delay  SampleTime=1
  cfblk2 : Outport
  wires:
  cfblk3/1 -> cfblk5/1
  cfblk1/1 -> cfblk2/1
  cfblk5/1 -> cfblk4/1
  cfblk4/1 -> cfblk6/1
  cfblk6/1 -> cfblk3/1
  cfblk5/2 -> cfblk7/1
  cfblk7/1 -> cfblk3/2

== system sampleModel281/cfblk90 ==
  cfblk1 : Inport
  cfblk3 : Inport  Port=2
  cfblk2 : Outport
  wires:
  cfblk3/1 -> cfblk2/1

== system sampleModel281/cfblk91 ==
  cfblk1 : Inport
  cfblk3 : Product  Inputs=*
  cfblk2 : Outport
  wires:
  cfblk1/1 -> cfblk3/1
  cfblk3/1 -> cfblk2/1

== system sampleModel281/cfblk92 ==
  cfblk1 : Inport
  cfblk3 : Sum  Inputs=-+
  cfblk2 : Outport
  wires:
  cfblk1/1 -> cfblk3/1, cfblk3/2
  cfblk3/1 -> cfblk2/1

== system sampleModel281/cfblk93 ==
  cfblk1 : Inport
  cfblk5 : Inport  Port=2
  cfblk3 : Abs
  cfblk4 : Product  Inputs=*
  cfblk2 : Outport
  wires:
  cfblk1/1 -> cfblk4/1
  cfblk5/1 -> cfblk2/1
  cfblk4/1 -> cfblk3/1

== system sampleModel281/cfblk94 ==
  cfblk1 : Inport
  cfblk3 : DiscreteFilter  SampleTime=1
  cfblk4 : Polyval  Coefs=[ +2.081618890e-019, -1.441693666e-014, +4.719686976e-010, -8.536869453e-006, +1.621573104e-001, -8.087801117e+001 ]
  cfblk5 : Constant  Value=[-730693865.910529]  SampleTime=1
  cfblk2 : Outport
  wires:
  cfblk1/1 -> cfblk3/1
  cfblk3/1 -> cfblk4/1
  cfblk5/1 -> cfblk2/1

== system sampleModel281/cfblk98 ==
  cfblk1 : Inport
  cfblk3 : Inport  Port=2
  Action Port : ActionPort  ActionPortLabel=if(u1 >= 0)
  cfblk2 : Outport
  wires:
  cfblk1/1 -> cfblk2/1

== system sampleModel281/cfblk99 ==
  cfblk1 : Inport
  Action Port : ActionPort  ActionPortLabel=else
  cfblk3 : DiscreteTransferFcn
  cfblk4 : Constant  Value=[173063756.286733]  SampleTime=1
  cfblk2 : Outport
  wires:
  cfblk1/1 -> cfblk3/1
  cfblk3/1 -> cfblk2/1
